simulink model "model"  (R2020b)
settings: Solver=VariableStepAuto  StartTime=0.0  StopTime=10.0  RelTol=1e-3
settings Model: Creator=Arvind Hishikar  LastModifiedBy=Arvind Hishikar

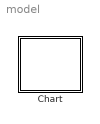
== system model ==
  Chart : Stateflow chart  TreatAsAtomicUnit=on

== stateflow chart model/Chart ==
